simulink model "BldcClosedLoop2"  (R2020b)
settings: Solver=ode45  StartTime=0.0  StopTime=1  FixedStep=.001  RelTol=1e-3  AbsTol=1e-3  EnableMultiTasking=on
values from neighbouring files (symbols this model uses):
  c1 = 3*wmax/(t1*t1)    (= 120000)    [data_bldc_ClosedLoop2.m]
  c2 = -2*wmax/(t1*t1*t1)    (= -800000)    [data_bldc_ClosedLoop2.m]
  D = 2e-3    (= 0.002)    [data_bldc_ClosedLoop2.m]
  d1 = 3*wmax/((t3-t2)*(t3-t2))    (= 120000)    [data_bldc_ClosedLoop2.m]
  d2 = -2*wmax/((t3-t2)*(t3-t2)*(t3-t2))    (= -800000)    [data_bldc_ClosedLoop2.m]
  ep = 0.5128    [data_bldc_ClosedLoop2.m]
  Gamma_Inv = Gamma^-1    [data_bldc_ClosedLoop2.m]
  J = 2.0e-4    (= 0.0002)    [data_bldc_ClosedLoop2.m]
  k0 = p0*p1*p2    (= 1000000)    [data_bldc_ClosedLoop2.m]
  k1 = p0*p1 + p0*p2 + p1*p2    (= 30000)    [data_bldc_ClosedLoop2.m]
  k2 = p0+p1+p2    (= 300)    [data_bldc_ClosedLoop2.m]
  KI = 0*1e6    (= 0)    [data_bldc_ClosedLoop2.m]
  Kp = 1000    [data_bldc_ClosedLoop2.m]
  Rs = 0.7    [data_bldc_ClosedLoop2.m]
  t3 = t2 + t1    (= 0.7)    [data_bldc_ClosedLoop2.m]
  tau_L = 0    [data_bldc_ClosedLoop2.m]
  tdd = .1    (= 0.1)    [data_bldc_ClosedLoop2.m]
libraries: simulink x2
(part 2 of 2)

== system BldcClosedLoop2/Controller/current commands/IS3c/0 < theta < 2pi ==
  theta : Inport
  Constant1 : Constant  Value=2*pi
  Fcn4 : Fcn  Expr=rem(u(1),2*pi)
  Scope1 : Scope
  Sum2 : Sum  Inputs=|++  InputSameDT=on  SaturateOnIntegerOverflow=on  OutDataTypeStr=Inherit: Same as first input
  Switch3 : Switch  SaturateOnIntegerOverflow=on  InputSameDT=on
  0 < theta < 2pi : Outport
  wires:
  Sum2/1 -> Switch3/3
  Fcn4/1 -> Sum2/1, Switch3/1, Switch3/2
  Constant1/1 -> Sum2/2
  theta/1 -> Fcn4/1, Scope1/1
  Switch3/1 -> 0 < theta < 2pi/1

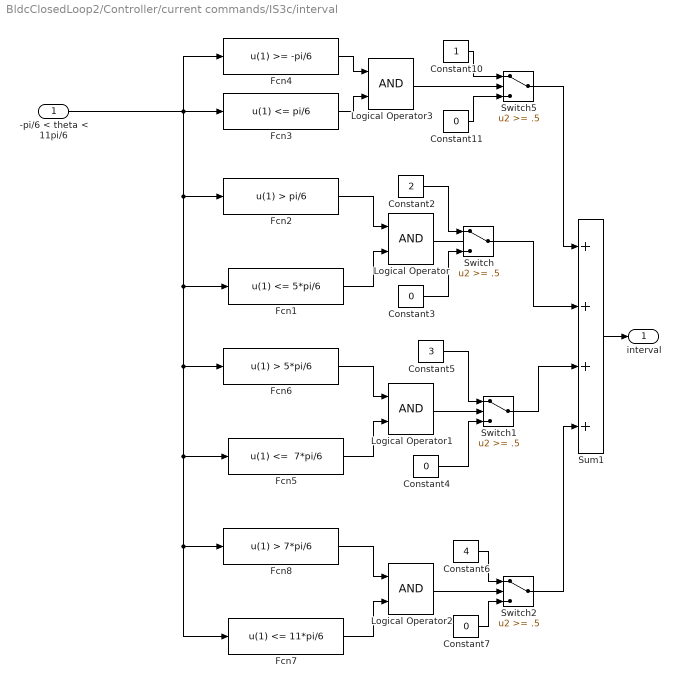
== system BldcClosedLoop2/Controller/current commands/IS3c/interval ==
  -pi/6 < theta < 11pi/6 : Inport
  Constant10 : Constant
  Constant{3..4,7,11} (4 alike) : Constant  Value=0
  Constant2 : Constant  Value=2
  Constant5 : Constant  Value=3
  Constant6 : Constant  Value=4
  Fcn1 : Fcn  Expr=u(1) <= 5*pi/6
  Fcn2 : Fcn  Expr=u(1) > pi/6
  Fcn3 : Fcn  Expr=u(1) <= pi/6
  Fcn4 : Fcn  Expr=u(1) >= -pi/6
  Fcn5 : Fcn  Expr="u(1) <=  7*pi/6"
  Fcn6 : Fcn  Expr=u(1) > 5*pi/6
  Fcn7 : Fcn  Expr=u(1) <= 11*pi/6
  Fcn8 : Fcn  Expr=u(1) > 7*pi/6
  Logical Operator{,1..3} (4 alike) : Logic
  Sum1 : Sum  Inputs=++++  InputSameDT=on  SaturateOnIntegerOverflow=on  OutDataTypeStr=Inherit: Same as first input
  Switch{,1..2,5} (4 alike) : Switch  Threshold=.5  SaturateOnIntegerOverflow=on  InputSameDT=on
  interval : Outport
  wires:
  Fcn1/1 -> Logical Operator/2
  Fcn2/1 -> Logical Operator/1
  Logical Operator/1 -> Switch/2
  Fcn5/1 -> Logical Operator1/2
  Fcn6/1 -> Logical Operator1/1
  Logical Operator1/1 -> Switch1/2
  Fcn7/1 -> Logical Operator2/2
  Fcn8/1 -> Logical Operator2/1
  Logical Operator2/1 -> Switch2/2
  Constant4/1 -> Switch1/3
  Constant10/1 -> Switch5/1
  Constant11/1 -> Switch5/3
  Switch1/1 -> Sum1/3
  Switch5/1 -> Sum1/1
  Constant2/1 -> Switch/1
  Constant5/1 -> Switch1/1
  Constant3/1 -> Switch/3
  Constant6/1 -> Switch2/1
  Constant7/1 -> Switch2/3
  Switch/1 -> Sum1/2
  Switch2/1 -> Sum1/4
  -pi/6 < theta < 11pi/6/1 -> Fcn3/1, Fcn2/1, Fcn1/1, Fcn6/1, Fcn5/1, Fcn8/1, Fcn7/1, Fcn4/1
  Sum1/1 -> interval/1
  Logical Operator3/1 -> Switch5/2
  Fcn4/1 -> Logical Operator3/1
  Fcn3/1 -> Logical Operator3/2
